simulink model "BLAC_MotorCtrl_Math"  (R2025b)
settings: Solver=FixedStepDiscrete  StartTime=0.0  StopTime=5  FixedStep=MC_Sim_BaseStep  RelTol=1e-3  EnableMultiTasking=on
values from neighbouring files (symbols this model uses):
  MC_Hardware_Chip_ADCResultBit = 0.0    [MotorControlDataDictionary_Math.sldd]
  MC_Hardware_Chip_ADCVoltageMax = 1.0    [MotorControlDataDictionary_Math.sldd]
  MC_Hardware_Chip_ADCVoltageRefence = 0.0    [MotorControlDataDictionary_Math.sldd]
  MC_Hardware_Chip_CSAGain = 1.0    [MotorControlDataDictionary_Math.sldd]
  MC_Sim_BaseStep = 2.5E-8    [MotorControlDataDictionary_Math.sldd]
  MC_Sim_HFTStep = 6.6675E-5    [MotorControlDataDictionary_Math.sldd]
undefined symbols (not defined in the file or in its folder): MC_MOS_DeadTime, MC_Motor_Phi, MC_Motor_Rotor_Pn, MC_Motor_Stator_Ld, MC_Motor_Stator_Lq, MC_Motor_Stator_Rs, MC_Param_CurrentPI_Ki, MC_Param_CurrentPI_Kp, MC_Param_CurrentPI_UdInteMax, MC_Param_CurrentPI_UdInteMin, MC_Param_CurrentPI_UdMax, MC_Param_CurrentPI_UdMin, MC_Param_CurrentPI_UqInteMax, MC_Param_CurrentPI_UqInteMin, MC_Param_CurrentPI_UqMax, MC_Param_CurrentPI_UqMin, MC_Param_Flux_Gamma, MC_Param_Flux_Lalpha, MC_Param_Flux_Lbeta, MC_Param_Flux_Ralpha, MC_Param_Flux_Rbeta, MC_Param_Luen_BEMFalpha, MC_Param_Luen_BEMFbeta, MC_Param_Luen_BEMFErr, MC_Param_Luen_Currentalpha, MC_Param_Luen_Currentbeta, MC_Param_Luen_CurrentErr, MC_Param_Luen_PLL_Ki, MC_Param_Luen_PLL_Kp, MC_Param_Luen_Voltagealpha, MC_Param_Luen_Voltagebeta, MC_Param_PhasetoReal, MC_Param_SMO_CoffA, MC_Param_SMO_CoffB, MC_Param_SpeedtoTheta, MC_Param_SVPWM_DutyMax, MC_Param_SVPWM_DutyMin, MC_Param_SVPWM_SampleOffset1, MC_Param_SVPWM_SampleOffset2, MC_Param_SVPWM_SampleValid
libraries: simulink x31, nesl_utility x22, ee_lib x21, fl_lib x16, spsSeriesRLCBranchLib x2, spsVoltageMeasurementLib x2
(part 4 of 5)

== system BLAC_MotorCtrl_Math/HFTask/fluxobservor/getFlux ==
  note: 日志：
      | 2025.02.28：滑膜观测器建模无问题，但是反电势观测存在问题，暂时分析为参数问题
  Valpha : Inport
  Vbeta : Inport  Port=2
  Ialpha : Inport  Port=3
  Ibeta : Inport  Port=4
  Add{,1..4} (5 alike) : Sum
  Constant : Constant  Value=MC_Motor_Phi  OutDataTypeStr=single
  Delay One Step{,1..3} (4 alike) : Delay  DelayLength=1
  Gain : Gain  Gain=MC_Param_Flux_Ralpha
  Gain1 : Gain  Gain=MC_Param_Flux_Gamma  OutDataTypeStr=single  RndMeth=Simplest
  Gain2 : Gain  Gain=single(MC_Sim_HFTStep)  OutDataTypeStr=single  RndMeth=Simplest
  Gain3 : Gain  Gain=MC_Param_Flux_Lalpha  OutDataTypeStr=single  RndMeth=Simplest
  Gain4 : Gain  Gain=MC_Param_Flux_Rbeta
  Gain5 : Gain  Gain=MC_Param_Flux_Gamma  OutDataTypeStr=single  RndMeth=Simplest
  Gain6 : Gain  Gain=single(MC_Sim_HFTStep)
  Gain7 : Gain  Gain=MC_Param_Flux_Lbeta  OutDataTypeStr=single  RndMeth=Simplest
  Product : Product
  Product1 : Product
  Square : Math  Operator=square
  Square1 : Math  Operator=square
  Square2 : Math  Operator=square
  Subtract{,1..4} (5 alike) : Sum  Inputs=+-
  Phialpha : Outport
  Phibeta : Outport  Port=2
  wires:
  Valpha/1 -> Subtract/1
  Ialpha/1 -> Gain3/1, Gain/1
  Gain/1 -> Subtract/2
  Subtract/1 -> Add/1  "Y_Alpha"
  Gain1/1 -> Add/2  "NLFcn_Alpha"
  Add/1 -> Gain2/1  "Xdot_Alpha"
  Add1/1 -> Subtract1/1, Delay One Step/1  "X_Alpha"
  Delay One Step/1 -> Add1/2
  Gain2/1 -> Add1/1
  Gain3/1 -> Subtract1/2
  Subtract1/1 -> Phialpha/1, Delay One Step1/1  "Phialpha"
  Product/1 -> Gain1/1
  Delay One Step1/1 -> [Nx_alpha], Product/2
  Delay One Step3/1 -> [Nx_beta], Product1/2
  Product1/1 -> Gain5/1
  Subtract3/1 -> Phibeta/1, Delay One Step3/1  "Phibeta"
  Gain7/1 -> Subtract3/2
  Gain6/1 -> Add3/1
  Delay One Step2/1 -> Add3/2
  Add3/1 -> Delay One Step2/1, Subtract3/1  "X_Beta"
  Add2/1 -> Gain6/1  "Xdot_Beta"
  Gain5/1 -> Add2/2  "NLFcn_Beta"
  Subtract2/1 -> Add2/1  "Y_Beta"
  Gain4/1 -> Subtract2/2
  Ibeta/1 -> Gain4/1, Gain7/1
  Vbeta/1 -> Subtract2/1
  Constant/1 -> Square/1
  [Nx_alpha] -> Square1/1
  [Nx_beta] -> Square2/1
  Square1/1 -> Add4/1
  Square2/1 -> Add4/2
  Square/1 -> Subtract4/1
  Add4/1 -> Subtract4/2  "Psim2"
  Subtract4/1 -> [Nx2]  "Nx2"
  [Nx2] -> Product/1
  [Nx2] -> Product1/1

== system BLAC_MotorCtrl_Math/HFTask/fluxobservor/getSpeedandTheta ==
  Phialpha : Inport
  Phibeta : Inport  Port=2
  Add : Sum
  Add1 : Sum
  Add2 : Sum
  Constant : Constant  Value=2*pi  OutDataTypeStr=single
  Delay One Step : Delay  DelayLength=1
  Delay One Step2 : Delay  DelayLength=1
  Gain : Gain  Gain=1/MC_Motor_Phi
  Gain1 : Gain  Gain=2*sqrt(2)/2*100
  Gain2 : Gain  Gain=100^2*MC_Sim_HFTStep
  Gain3 : Gain  Gain=MC_Param_SpeedtoTheta  OutDataTypeStr=single  RndMeth=Simplest
  Gain4 : Gain  Gain=1/MC_Motor_Phi
  Gain5 : Gain  Gain=30/(pi*MC_Motor_Rotor_Pn)  OutDataTypeStr=single  RndMeth=Simplest
  Mod : Math  Operator=mod
  Product : Product
  Product1 : Product
  Sin : Trigonometry  OutputSignalType=real
  Sin1 : Trigonometry  Operator=cos  OutputSignalType=real
  Subtract : Sum  Inputs=+-
  Speed : Outport
  Theta : Outport  Port=2
  wires:
  [Theta_Last] -> Sin/1, Sin1/1
  Add1/1 -> Gain5/1, Gain3/1  "WeFlux"
  Mod/1 -> Delay One Step2/1, Theta/1  "ThetaFlux"
  Delay One Step2/1 -> [Theta_Last], Add2/2
  Constant/1 -> Mod/2
  Add2/1 -> Mod/1
  Gain3/1 -> Add2/1
  Subtract/1 -> Gain1/1, Gain2/1  "FluxErr"
  Gain1/1 -> Add1/1
  Delay One Step/1 -> Add/2
  Add/1 -> Add1/2, Delay One Step/1
  Gain2/1 -> Add/1
  Product1/1 -> Subtract/2  "FluxSin"
  Product/1 -> Subtract/1  "FluxCos"
  Sin/1 -> Product1/2
  Sin1/1 -> Product/2
  Phibeta/1 -> Gain/1
  Phialpha/1 -> Gain4/1
  Gain/1 -> Product/1
  Gain4/1 -> Product1/1
  Gain5/1 -> Speed/1  "SpeedFlux_RPM"

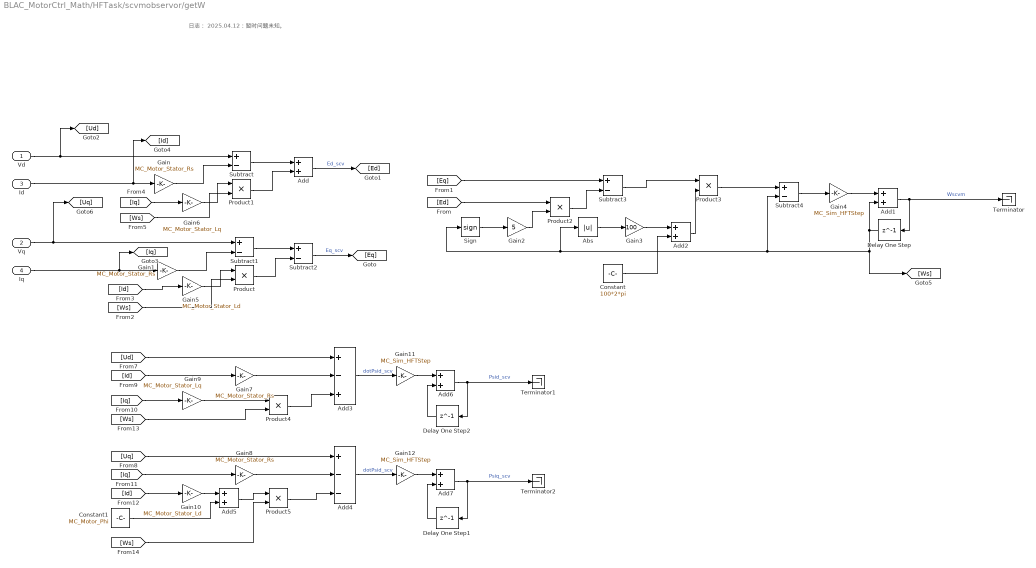
== system BLAC_MotorCtrl_Math/HFTask/scvmobservor/getW ==
  note: 日志：
      | 2025.04.12：暂时问题未知。
  Vd : Inport
  Vq : Inport  Port=2
  Id : Inport  Port=3
  Iq : Inport  Port=4
  Abs : Abs  SaturateOnIntegerOverflow=off
  Add{,1..2,5..7} (6 alike) : Sum
  Add3 : Sum  Inputs=+-+
  Add4 : Sum  Inputs=+--
  Constant : Constant  Value=100*2*pi  OutDataTypeStr=single
  Constant1 : Constant  Value=MC_Motor_Phi  OutDataTypeStr=single
  Delay One Step : Delay  DelayLength=1
  Delay One Step1 : Delay  DelayLength=1
  Delay One Step2 : Delay  DelayLength=1
  Gain{,1,7..8} (4 alike) : Gain  Gain=MC_Motor_Stator_Rs
  Gain10 : Gain  Gain=MC_Motor_Stator_Ld
  Gain11 : Gain  Gain=MC_Sim_HFTStep
  Gain12 : Gain  Gain=MC_Sim_HFTStep
  Gain2 : Gain  Gain=5
  Gain3 : Gain  Gain=100
  Gain4 : Gain  Gain=MC_Sim_HFTStep
  Gain5 : Gain  Gain=MC_Motor_Stator_Ld
  Gain6 : Gain  Gain=MC_Motor_Stator_Lq
  Gain9 : Gain  Gain=MC_Motor_Stator_Lq
  Product{,1..5} (6 alike) : Product
  Sign : Signum
  Subtract{,1..4} (5 alike) : Sum  Inputs=+-
  Terminator : Terminator
  Terminator1 : Terminator
  Terminator2 : Terminator
  wires:
  Id/1 -> [Id], Gain/1
  Gain/1 -> Subtract/2
  Subtract/1 -> Add/1
  Add/1 -> [Ed]  "Ed_scv"
  Gain1/1 -> Subtract1/2
  Iq/1 -> [Iq], Gain1/1
  Vq/1 -> Subtract1/1, [Uq]
  Subtract1/1 -> Subtract2/1
  Product/1 -> Subtract2/2
  Product1/1 -> Add/2
  Subtract2/1 -> [Eq]  "Eq_scv"
  [Ed] -> Product2/1
  Gain2/1 -> Product2/2
  Sign/1 -> Gain2/1
  [Eq] -> Subtract3/1
  Product2/1 -> Subtract3/2
  Subtract3/1 -> Product3/1
  Product3/1 -> Subtract4/1
  Gain4/1 -> Add1/1
  Add1/1 -> Delay One Step/1, Terminator/1  "Wscvm"
  Delay One Step/1 -> [Ws], Subtract4/2, Abs/1, Sign/1, Add1/2
  Subtract4/1 -> Gain4/1
  [Id] -> Gain5/1
  Gain5/1 -> Product/1
  [Ws] -> Product/2
  Gain6/1 -> Product1/1
  [Iq] -> Gain6/1
  [Ws] -> Product1/2
  Abs/1 -> Gain3/1
  Add2/1 -> Product3/2
  Gain3/1 -> Add2/1
  Constant/1 -> Add2/2
  Vd/1 -> Subtract/1, [Ud]
  [Id] -> Gain7/1
  [Iq] -> Gain8/1
  [Ud] -> Add3/1
  Gain7/1 -> Add3/2
  Gain8/1 -> Add4/2
  [Uq] -> Add4/1
  [Ws] -> Product4/2
  Product4/1 -> Add3/3
  Product5/1 -> Add4/3
  [Iq] -> Gain9/1
  Gain9/1 -> Product4/1
  [Id] -> Gain10/1
  Gain10/1 -> Add5/1
  Constant1/1 -> Add5/2
  Add5/1 -> Product5/1
  [Ws] -> Product5/2
  Add3/1 -> Gain11/1  "dotPsid_scv"
  Add4/1 -> Gain12/1  "dotPsid_scv"
  Add7/1 -> Terminator2/1, Delay One Step1/1  "Psiq_scv"
  Delay One Step1/1 -> Add7/2
  Add6/1 -> Terminator1/1, Delay One Step2/1  "Psid_scv"
  Delay One Step2/1 -> Add6/2
  Gain11/1 -> Add6/1
  Gain12/1 -> Add7/1

== system BLAC_MotorCtrl_Math/HFTask/smo/getE ==
  note: 日志：
      | 2025.02.28：滑膜观测器建模无问题，但是反电势观测存在问题，暂时分析为参数问题
  Valpha : Inport
  Vbeta : Inport  Port=2
  Ialpha : Inport  Port=3
  Ibeta : Inport  Port=4
  Add : Sum  Inputs=--+
  Add1 : Sum
  Add2 : Sum  Inputs=+--
  Add3 : Sum
  Delay One Step{,1..3} (4 alike) : Delay  DelayLength=1
  Gain{,4,6,8} (4 alike) : Gain  Gain=MC_Param_SMO_CoffB
  Gain3 : Gain  Gain=MC_Param_SMO_CoffA
  Gain7 : Gain  Gain=MC_Param_SMO_CoffA
  Saturation : Saturate  UpperLimit=100  LowerLimit=-100
  Saturation1 : Saturate  UpperLimit=100  LowerLimit=-100
  Subtract : Sum  Inputs=+-
  Subtract1 : Sum  Inputs=-+
  Ealpha : Outport
  Ebeta : Outport  Port=2
  wires:
  Valpha/1 -> Gain/1
  Add1/1 -> Subtract/1, Delay One Step/1  "Ialpha_SMO"
  Ialpha/1 -> Subtract/2
  Gain/1 -> Add/3
  Gain3/1 -> Add/2
  Gain4/1 -> Add/1
  Delay One Step1/1 -> [Ealpha_SMO]
  [Ialpha_SMO] -> Gain3/1
  [Ealpha_SMO] -> Gain4/1
  Subtract/1 -> Saturation/1
  Saturation/1 -> Ealpha/1, Delay One Step1/1  "Ealpha_SMO"
  Gain6/1 -> Add2/1
  Gain7/1 -> Add2/2
  Gain8/1 -> Add2/3
  Vbeta/1 -> Gain6/1
  Add/1 -> Add1/1  "dotIalpha_SMO"
  Delay One Step/1 -> Add1/2, [Ialpha_SMO]
  Add2/1 -> Add3/2  "dotIbeta_SMO"
  Add3/1 -> Subtract1/2, Delay One Step2/1  "Ibeta_SMO"
  Delay One Step2/1 -> [Ibeta_SMO], Add3/1
  Ibeta/1 -> Subtract1/1
  Subtract1/1 -> Saturation1/1
  Saturation1/1 -> Ebeta/1, Delay One Step3/1  "Ebeta_SMO"
  Delay One Step3/1 -> [Ebeta_SMO]
  [Ibeta_SMO] -> Gain7/1
  [Ebeta_SMO] -> Gain8/1

== system BLAC_MotorCtrl_Math/HFTask/smo/getSpeedandTheta ==
  note: 日志：
      | 2025.03.19：反电势正负号识别错误，改正后可以使用
  Ealpha : Inport
  Ebeta : Inport  Port=2
  Add : Sum
  Add1 : Sum
  Add2 : Sum
  Constant : Constant  Value=2*pi  OutDataTypeStr=single
  Delay One Step : Delay  DelayLength=1
  Delay One Step2 : Delay  DelayLength=1
  Gain : Gain  Gain=-1
  Gain1 : Gain  Gain=2*sqrt(2)/2*100
  Gain2 : Gain  Gain=100^2*MC_Sim_HFTStep
  Gain3 : Gain  Gain=MC_Param_SpeedtoTheta
  Gain5 : Gain  Gain=30/(pi*MC_Motor_Rotor_Pn)  OutDataTypeStr=single  RndMeth=Simplest
  Mod : Math  Operator=mod
  Product : Product
  Product1 : Product
  Sin : Trigonometry  OutputSignalType=real
  Sin1 : Trigonometry  Operator=cos  OutputSignalType=real
  Subtract : Sum  Inputs=+-
  Speed : Outport
  Theta : Outport  Port=2
  wires:
  Sin1/1 -> Product/2
  Sin/1 -> Product1/2
  Gain2/1 -> Add/1
  Add/1 -> Delay One Step/1, Add1/2
  Delay One Step/1 -> Add/2
  Gain1/1 -> Add1/1
  Subtract/1 -> Gain2/1, Gain1/1  "SMOErr"
  Gain3/1 -> Add2/1
  Add2/1 -> Mod/1
  Constant/1 -> Mod/2
  Delay One Step2/1 -> Add2/2, [Theta_Last]
  Mod/1 -> Theta/1, Delay One Step2/1  "ThetaSMO"
  Add1/1 -> Gain5/1, Gain3/1  "SpeedSmo"
  [Theta_Last] -> Sin1/1, Sin/1
  Gain/1 -> Product1/1
  Ebeta/1 -> Gain/1
  Ealpha/1 -> Product/1
  Product/1 -> Subtract/1  "SMOSin"
  Product1/1 -> Subtract/2  "SMOCos"
  Gain5/1 -> Speed/1  "SpeedSMO_RPM"

== system BLAC_MotorCtrl_Math/HFTask/svpwm/getVoltageExchange ==
  Valpha : Inport
  Vbeta : Inport  Port=2
  Vdc : Inport  Port=3
  Add : Sum
  Add1 : Sum
  Divide : Product  Inputs=*/
  Divide1 : Product  Inputs=*/
  Gain : Gain  Gain=-1/2
  Gain1 : Gain  Gain=sqrt(3)/2
  Gain2 : Gain  Gain=-1
  Relational Operator : RelationalOperator  OutDataTypeStr=boolean  RndMeth=Simplest  InputSameDT=off
  Relational Operator1 : RelationalOperator  OutDataTypeStr=boolean  RndMeth=Simplest  InputSameDT=off
  Relational Operator2 : RelationalOperator  Operator=<=  OutDataTypeStr=boolean  RndMeth=Simplest  InputSameDT=off
  Relational Operator3 : RelationalOperator  Operator=<=  OutDataTypeStr=boolean  RndMeth=Simplest  InputSameDT=off
  Signal Copy : SignalConversion  OverrideOpt=off
  Subtract : Sum  Inputs=+-
  Switch{,1..3} (4 alike) : Switch  Criteria=u2 > Threshold  SaturateOnIntegerOverflow=off  InputSameDT=off
  getSectorN : Subsystem  Commented=on
  Va : Outport
  Vb : Outport  Port=2
  Vc : Outport  Port=3
  Vmed : Outport  Port=4
  wires:
  Valpha/1 -> Divide/1
  Vbeta/1 -> Divide1/1
  Vdc/1 -> Divide/2, Divide1/2
  Subtract/1 -> Relational Operator3/2, Switch3/3, Relational Operator1/2, Switch1/3, Vc/1  "Vc"
  Add/1 -> Switch2/3, Relational Operator2/2, Switch/3, Relational Operator/2, Vb/1  "Vb"
  Gain1/1 -> Subtract/2, Add/2
  Gain/1 -> Add/1, Subtract/1
  Divide1/1 -> Gain1/1
  Divide/1 -> Gain/1, Signal Copy/1
  Signal Copy/1 -> Switch2/1, Relational Operator2/1, Switch/1, Relational Operator/1, Va/1  "Va"
  Switch1/1 -> Add1/1  "Vmax"
  Relational Operator1/1 -> Switch1/2
  Switch/1 -> Relational Operator1/1, Switch1/1
  Relational Operator/1 -> Switch/2
  Switch3/1 -> Add1/2  "Vmin"
  Relational Operator3/1 -> Switch3/2
  Switch2/1 -> Switch3/1, Relational Operator3/1
  Relational Operator2/1 -> Switch2/2
  Add1/1 -> Gain2/1
  Gain2/1 -> Vmed/1  "Vmed"

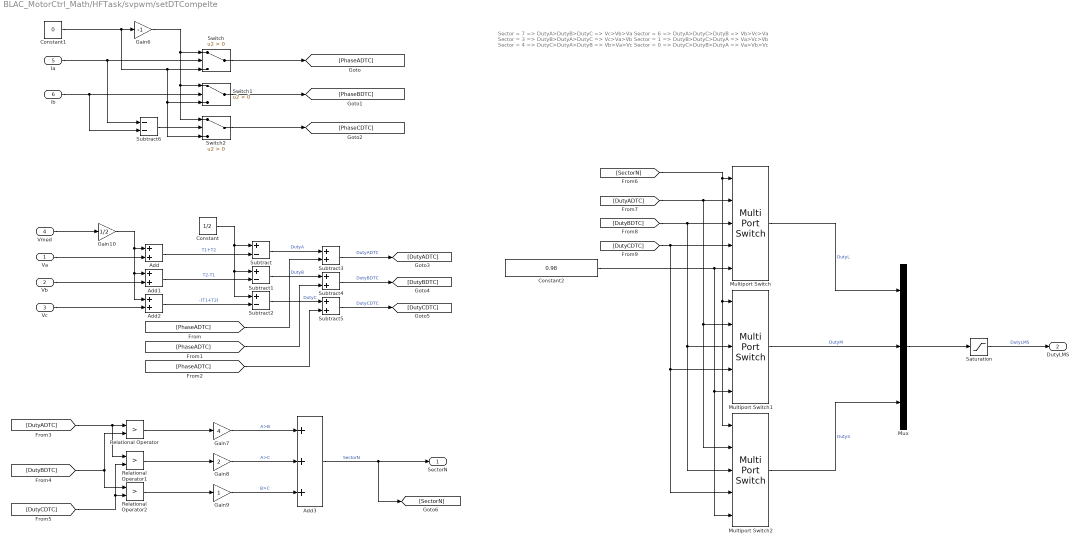
== system BLAC_MotorCtrl_Math/HFTask/svpwm/setDTCompelte ==
  note: Sector = 7 => DutyA>DutyB>DutyC => Vc>Vb>Va
      | Sector = 6 => DutyA>DutyC>DutyB => Vb>Vc>Va
      | Sector = 3 => DutyB>DutyA>DutyC => Vc>Va>Vb
      | Sector = 1 => DutyB>DutyC>DutyA => Va>Vc>Vb
      | Sector = 4 => DutyC>DutyA>DutyB => Vb>Va>Vc
      | Sector = 0 => DutyC>DutyB>DutyA => Va>Vb>Vc
  Va : Inport
  Vb : Inport  Port=2
  Vc : Inport  Port=3
  Vmed : Inport  Port=4
  Ia : Inport  Port=5
  ib : Inport  Port=6
  Add : Sum
  Add1 : Sum
  Add2 : Sum
  Add3 : Sum  Inputs=+++
  Constant : Constant  Value=1/2  OutDataTypeStr=single  SampleTime=MC_Sim_HFTStep
  Constant1 : Constant  Value=0  OutDataTypeStr=single
  Constant2 : Constant  Value=0.98  OutDataTypeStr=single
  Gain10 : Gain  Gain=1/2
  Gain6 : Gain  Gain=-1
  Gain7 : Gain  Gain=4  OutDataTypeStr=single  RndMeth=Simplest
  Gain8 : Gain  Gain=2  OutDataTypeStr=single  RndMeth=Simplest
  Gain9 : Gain  OutDataTypeStr=single  RndMeth=Simplest
  Multiport Switch : MultiPortSwitch  DataPortOrder=Specify indices  DataPortIndices={[6,7],[1,3],[0,4]}  DataPortForDefault=Additional data port  SaturateOnIntegerOverflow=off  InputSameDT=off
  Multiport Switch1 : MultiPortSwitch  DataPortOrder=Specify indices  DataPortIndices={[4,3],[7,0],[6,1]}  DataPortForDefault=Additional data port  SaturateOnIntegerOverflow=off  InputSameDT=off
  Multiport Switch2 : MultiPortSwitch  DataPortOrder=Specify indices  DataPortIndices={[0,1],[4,6],[3,7]}  DataPortForDefault=Additional data port  SaturateOnIntegerOverflow=off  InputSameDT=off
  Mux : Mux  Inputs=3
  Relational Operator : RelationalOperator  Operator=>  OutDataTypeStr=boolean  RndMeth=Simplest  InputSameDT=off
  Relational Operator1 : RelationalOperator  Operator=>  OutDataTypeStr=boolean  RndMeth=Simplest  InputSameDT=off
  Relational Operator2 : RelationalOperator  Operator=>  OutDataTypeStr=boolean  RndMeth=Simplest  InputSameDT=off
  Saturation : Saturate  UpperLimit=0.98  LowerLimit=0.02
      settings: AttributesFormatString=|
      | OutputMax = %<UpperLimit>
      | OutputMin = %<LowerLimit>
  Subtract : Sum  Inputs=+-
  Subtract1 : Sum  Inputs=+-
  Subtract2 : Sum  Inputs=+-
  Subtract3 : Sum
  Subtract4 : Sum
  Subtract5 : Sum
  Subtract6 : Sum  Inputs=--
  Switch : Switch  Criteria=u2 > Threshold  SaturateOnIntegerOverflow=off  InputSameDT=off
  Switch1 : Switch  Criteria=u2 > Threshold  SaturateOnIntegerOverflow=off  InputSameDT=off
  Switch2 : Switch  Criteria=u2 > Threshold  SaturateOnIntegerOverflow=off  InputSameDT=off
  SectorN : Outport
  DutyLMS : Outport  Port=2
  wires:
  Va/1 -> Add/2
  Vmed/1 -> Gain10/1
  Vb/1 -> Add1/2
  Vc/1 -> Add2/2
  Add/1 -> Subtract/2  "T1+T2"
  Add2/1 -> Subtract2/2  "-(T1+T2)"
  Add1/1 -> Subtract1/2  "T2-T1"
  Constant/1 -> Subtract2/1, Subtract1/1, Subtract/1
  Subtract/1 -> Subtract3/1  "DutyA"
  Subtract1/1 -> Subtract4/1  "DutyB"
  Subtract2/1 -> Subtract5/1  "DutyC"
  Ia/1 -> Subtract6/1, Switch/2
  Gain6/1 -> Switch2/1, Switch1/1, Switch/1
  ib/1 -> Subtract6/2, Switch1/2
  Subtract6/1 -> Switch2/2
  Constant1/1 -> Switch2/3, Switch1/3, Switch/3, Gain6/1
  Switch/1 -> [PhaseADTC]
  Switch1/1 -> [PhaseBDTC]
  Switch2/1 -> [PhaseCDTC]
  [PhaseADTC] -> Subtract3/2
  [PhaseADTC] -> Subtract4/2
  [PhaseADTC] -> Subtract5/2
  [DutyBDTC] -> Relational Operator/2, Relational Operator2/1
  [DutyADTC] -> Relational Operator1/1, Relational Operator/1
  [DutyCDTC] -> Relational Operator2/2, Relational Operator1/2
  Relational Operator/1 -> Gain7/1
  Relational Operator1/1 -> Gain8/1
  Relational Operator2/1 -> Gain9/1
  Gain8/1 -> Add3/2  "A>C"
  Gain9/1 -> Add3/3  "B>C"
  Gain7/1 -> Add3/1  "A>B"
  Add3/1 -> [SectorN], SectorN/1  "SectorN"
  Gain10/1 -> Add2/1, Add1/1, Add/1
  Subtract3/1 -> [DutyADTC]  "DutyADTC"
  Subtract4/1 -> [DutyBDTC]  "DutyBDTC"
  Subtract5/1 -> [DutyCDTC]  "DutyCDTC"
  [SectorN] -> Multiport Switch2/1, Multiport Switch1/1, Multiport Switch/1
  Multiport Switch/1 -> Mux/1  "DutyL"
  Constant2/1 -> Multiport Switch2/5, Multiport Switch1/5, Multiport Switch/5
  Multiport Switch1/1 -> Mux/2  "DutyM"
  Multiport Switch2/1 -> Mux/3  "DutyS"
  Mux/1 -> Saturation/1
  Saturation/1 -> DutyLMS/1  "DutyLMS"
  [DutyADTC] -> Multiport Switch2/2, Multiport Switch1/2, Multiport Switch/2
  [DutyCDTC] -> Multiport Switch2/4, Multiport Switch1/4, Multiport Switch/4
  [DutyBDTC] -> Multiport Switch2/3, Multiport Switch1/3, Multiport Switch/3

== system BLAC_MotorCtrl_Math/HFTask/svpwm/setPhaseandSample_ORS_Double ==
  note: 电流采样方案：
      | 1、电压满足采样时间，直接计算电流采样点，采样点有效
      | 2、周期内总电压满足采样时间，
  note: Sector = 7 => DutyA>DutyB>DutyC => Vc>Vb>Va
      | Sector = 6 => DutyA>DutyC>DutyB => Vb>Vc>Va
      | Sector = 3 => DutyB>DutyA>DutyC => Vc>Va>Vb
      | Sector = 1 => DutyB>DutyC>DutyA => Va>Vc>Vb
      | Sector = 4 => DutyC>DutyA>DutyB => Vb>Va>Vc
      | Sector = 0 => DutyC>DutyB>DutyA => Va>Vb>Vc
  SectorN : Inport
  DutyLMS : Inport  Port=2
  Constant{1,4,6..8} (5 alike) : Constant  OutDataTypeStr=single
  Constant2 : Constant  Value=boolean(1)  OutDataTypeStr=single
  Constant3 : Constant  Value=boolean(1)  OutDataTypeStr=single
  Constant5 : Constant  Value=0.98  OutDataTypeStr=single
  Demux : Demux  Outputs=3
  Multiport Switch : MultiPortSwitch  DataPortOrder=Specify indices  DataPortIndices={[7,6],[3,4],[0,1]}  DataPortForDefault=Additional data port  SaturateOnIntegerOverflow=off  InputSameDT=off
  Multiport Switch1 : MultiPortSwitch  DataPortOrder=Specify indices  DataPortIndices={[3,1],[7,0],[6,4]}  DataPortForDefault=Additional data port  SaturateOnIntegerOverflow=off  InputSameDT=off
  Multiport Switch2 : MultiPortSwitch  DataPortOrder=Specify indices  DataPortIndices={[4,0],[6,1],[7,3]}  DataPortForDefault=Additional data port  SaturateOnIntegerOverflow=off  InputSameDT=off
  Mux : Mux  Inputs=2
  Mux1 : Mux  Inputs=5
  Mux2 : Mux  Inputs=2
  Mux5 : Mux  Inputs=3
  Saturation : Saturate  UpperLimit=0.98  LowerLimit=0.02
      settings: AttributesFormatString=|
      | OutputMax = %<UpperLimit>
      | OutputMin = %<LowerLimit>
  Subtract : Sum  Inputs=+-
  Subtract1 : Sum  Inputs=+-
  DutySVPWM : Outport
  SamplePoint : Outport  Port=2
  SampleValid : Outport  Port=3
  wires:
  DutyLMS/1 -> Demux/1
  Subtract/1 -> [T1divid2]  "T1/2"
  Subtract1/1 -> [T2divid2]  "T2/2"
  SectorN/1 -> [SectorN]
  [SectorN] -> Multiport Switch2/1, Multiport Switch1/1, Multiport Switch/1
  [DutyLPM] -> Multiport Switch2/2, Multiport Switch1/2, Multiport Switch/2
  [DutyMPM] -> Multiport Switch2/3, Multiport Switch1/3, Multiport Switch/3
  [DutySPM] -> Multiport Switch1/4, Multiport Switch2/4, Multiport Switch/4
  Constant5/1 -> Multiport Switch1/5, Multiport Switch/5, Multiport Switch2/5
  Multiport Switch1/1 -> Mux5/2  "DutyBPM[2]"
  Multiport Switch2/1 -> Mux5/3  "DutyCPM[2]"
  Multiport Switch/1 -> Mux5/1  "DutyAPM[2]"
  Saturation/1 -> DutySVPWM/1  "DutySVPWM[6]"
  Demux/1 -> [DutyL], Subtract1/1
  Demux/2 -> [DutyM], Subtract1/2, Subtract/1
  Demux/3 -> Subtract/2, [DutyS]
  Constant2/1 -> Mux/1
  Constant3/1 -> Mux/2
  Mux/1 -> SampleValid/1
  Constant4/1 -> Mux1/2
  Constant1/1 -> Mux1/1
  Mux1/1 -> SamplePoint/1
  Constant6/1 -> Mux1/3
  Constant8/1 -> Mux1/4
  Constant7/1 -> Mux1/5
  Mux5/1 -> Mux2/2, Mux2/1
  Mux2/1 -> Saturation/1

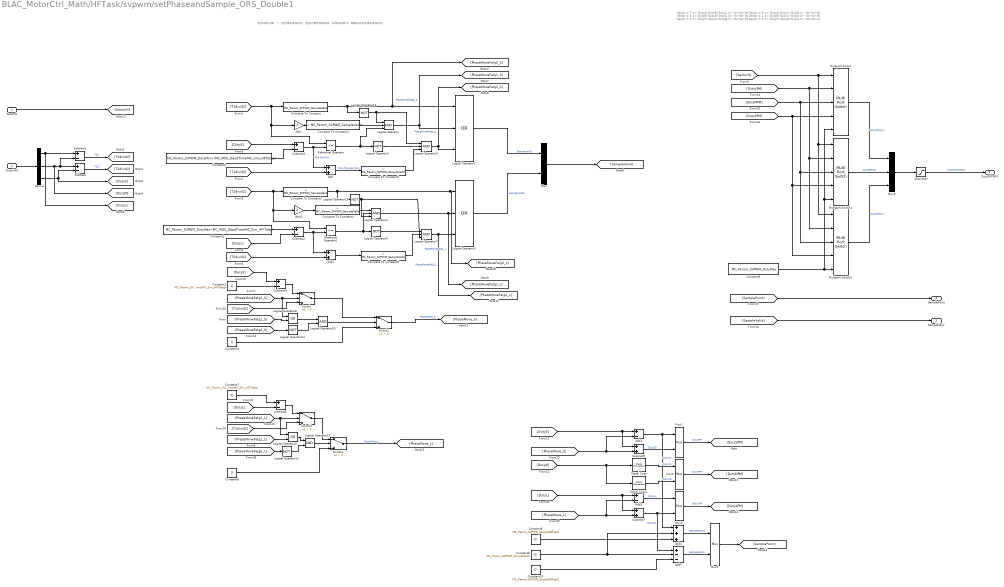
== system BLAC_MotorCtrl_Math/HFTask/svpwm/setPhaseandSample_ORS_Double1 ==
  note: Sector = 7 => DutyA>DutyB>DutyC => Vc>Vb>Va
      | Sector = 6 => DutyA>DutyC>DutyB => Vb>Vc>Va
      | Sector = 3 => DutyB>DutyA>DutyC => Vc>Va>Vb
      | Sector = 1 => DutyB>DutyC>DutyA => Va>Vc>Vb
      | Sector = 4 => DutyC>DutyA>DutyB => Vb>Va>Vc
      | Sector = 0 => DutyC>DutyB>DutyA => Va>Vb>Vc
  note: 电流采样方案：
      | 1、电压满足采样时间，直接计算电流采样点，采样点有效
      | 2、周期内总电压满足采样时间，
  SectorN : Inport
  DutyLMS : Inport  Port=2
  Add : Sum
  Add1 : Sum
  Add2 : Sum  Inputs=+-
  Add3 : Sum  Inputs=+-
  Add4 : Sum  Inputs=+++
  Add5 : Sum  Inputs=+--
  Compare To Constant{,1..5} (6 alike) : simulink/Logic and Bit Operations/Compare To Constant  relop=>  const=MC_Param_SVPWM_SampleValid  OutDataTypeStr=boolean
  Constant1 : Constant  Value=MC_Param_SVPWM_DutyMax-(MC_MOS_DeadTime/MC_Sim_HFTStep)  OutDataTypeStr=single
  Constant10 : Constant  Value=MC_Param_SVPWM_SampleOffset2  OutDataTypeStr=single
  Constant2 : Constant  Value=MC_Param_SVPWM_DutyMin+(MC_MOS_DeadTime/MC_Sim_HFTStep)  OutDataTypeStr=single
  Constant3 : Constant  Value=MC_Param_SVPWM_DutyMin+(MC_MOS_DeadTime/MC_Sim_HFTStep)  OutDataTypeStr=single
  Constant4 : Constant  Value=0  OutDataTypeStr=single
  Constant5 : Constant  Value=MC_Param_SVPWM_DutyMax  OutDataTypeStr=single
  Constant6 : Constant  Value=0  OutDataTypeStr=single
  Constant7 : Constant  Value=MC_Param_SVPWM_DutyMax-(MC_MOS_DeadTime/MC_Sim_HFTStep)  OutDataTypeStr=single
  Constant8 : Constant  Value=MC_Param_SVPWM_SampleValid  OutDataTypeStr=single
  Constant9 : Constant  Value=MC_Param_SVPWM_SampleOffset1  OutDataTypeStr=single
  Demux : Demux  Outputs=3
  Gain : Gain  Gain=2
  Gain1 : Gain  Gain=2
  Logical Operator{,3..4,7} (4 alike) : Logic  Inputs=3  AllPortsSameDT=off  OutDataTypeStr=boolean
  Logical Operator1 : Logic  Operator=OR  Inputs=3  AllPortsSameDT=off  OutDataTypeStr=boolean
  Logical Operator10 : Logic  AllPortsSameDT=off  OutDataTypeStr=boolean
  Logical Operator{2,6,11..12,14..15} (6 alike) : Logic  Operator=NOT  AllPortsSameDT=off  OutDataTypeStr=boolean
  Logical Operator13 : Logic  AllPortsSameDT=off  OutDataTypeStr=boolean
  Logical Operator5 : Logic  Operator=OR  Inputs=3  AllPortsSameDT=off  OutDataTypeStr=boolean
  Logical Operator8 : Logic  Operator=OR  AllPortsSameDT=off  OutDataTypeStr=boolean
  Logical Operator9 : Logic  Operator=OR  AllPortsSameDT=off  OutDataTypeStr=boolean
  Multiport Switch : MultiPortSwitch  DataPortOrder=Specify indices  DataPortIndices={[7,6],[3,4],[0,1]}  DataPortForDefault=Additional data port  SaturateOnIntegerOverflow=off  InputSameDT=off
  Multiport Switch1 : MultiPortSwitch  DataPortOrder=Specify indices  DataPortIndices={[3,1],[7,0],[6,4]}  DataPortForDefault=Additional data port  SaturateOnIntegerOverflow=off  InputSameDT=off
  Multiport Switch2 : MultiPortSwitch  DataPortOrder=Specify indices  DataPortIndices={[4,0],[6,1],[7,3]}  DataPortForDefault=Additional data port  SaturateOnIntegerOverflow=off  InputSameDT=off
  Mux{,1..4} (5 alike) : Mux  Inputs=2
  Mux5 : Mux  Inputs=3
  Relational Operator : RelationalOperator  Operator=<=  OutDataTypeStr=boolean  RndMeth=Simplest  InputSameDT=off
  Relational Operator1 : RelationalOperator  Operator=<=  OutDataTypeStr=boolean  RndMeth=Simplest  InputSameDT=off
  Saturation : Saturate  UpperLimit=MC_Param_SVPWM_DutyMax  LowerLimit=MC_Param_SVPWM_DutyMin
      settings: AttributesFormatString=|
      | OutputMax = %<UpperLimit>
      | OutputMin = %<LowerLimit>
  Signal Copy : SignalConversion  OverrideOpt=off
  Signal Copy1 : SignalConversion  OverrideOpt=off
  Subtract{,1..4,6} (6 alike) : Sum  Inputs=+-
  Subtract5 : Sum
  Subtract7 : Sum
  Switch{,1..3} (4 alike) : Switch  Criteria=u2 > Threshold  SaturateOnIntegerOverflow=off  InputSameDT=off
  DutySVPWM : Outport
  SamplePoint : Outport  Port=2
  SampleValid : Outport  Port=3
  wires:
  Logical Operator15/1 -> Logical Operator7/3, Logical Operator4/3
  Compare To Constant2/1 -> Logical Operator3/3
  Logical Operator2/1 -> Logical Operator3/2
  Logical Operator14/1 -> Logical Operator/1, Logical Operator3/1
  Compare To Constant1/1 -> Logical Operator/2
  Logical Operator12/1 -> Logical Operator13/2
  Logical Operator9/1 -> Logical Operator13/1
  Logical Operator13/1 -> Switch2/2
  [PhaseMoveFalg0_L] -> Logical Operator12/1
  [PhaseMoveFalg1_S] -> Logical Operator8/2
  Logical Operator11/1 -> Logical Operator10/2
  [PhaseMoveFalg0_S] -> Logical Operator11/1
  Logical Operator8/1 -> Logical Operator10/1
  Logical Operator10/1 -> Switch1/2
  [PhaseMoveFalg1_L] -> Logical Operator9/2
  [PhaseMoveFalg2_L] -> Switch3/2, Logical Operator9/1
  Constant10/1 -> Add5/3
  Constant9/1 -> Add4/3
  Mux4/1 -> [SamplePoint]
  Add5/1 -> Mux4/2  "SamplePoint2"
  Add4/1 -> Mux4/1  "SamplePoint1"
  Constant8/1 -> Add5/2, Add4/2
  Mux3/1 -> [DutyMPM]  "DutyMPM"
  Mux2/1 -> [DutyLPM]  "DutyLPM"
  Mux1/1 -> [DutySPM]  "DutySPM"
  Signal Copy/1 -> Mux3/1  "DutyMU"
  Signal Copy1/1 -> Mux3/2  "DutyMD"
  [DutyM] -> Signal Copy/1, Signal Copy1/1
  [DutyL] -> Subtract7/1, Add3/1
  [PhaseMove_L] -> Add3/2, Subtract7/2
  Add3/1 -> Mux2/1  "DutyLU"
  Subtract7/1 -> Mux2/2, Add5/1  "DutyLD"
  Subtract5/1 -> Mux1/2  "DutySD"
  Add2/1 -> Add4/1, Mux1/1  "DutySU"
  [PhaseMove_S] -> Subtract5/2, Add2/2
  [DutyS] -> Add2/1, Subtract5/1
  Demux/3 -> [DutyS], Subtract/2
  Demux/2 -> Subtract/1, Subtract1/2, [DutyM]
  Demux/1 -> Subtract1/1, [DutyL]
  Subtract6/1 -> Switch3/1
  Constant7/1 -> Subtract6/1
  [DutyL] -> Subtract6/2
  Switch3/1 -> Switch2/1
  [T2divid2] -> Switch3/3
  Constant6/1 -> Switch2/3
  Switch2/1 -> [PhaseMove_L]  "PhaseMove_L"
  Subtract4/1 -> Switch/1
  [T1divid2] -> Switch/3
  Switch1/1 -> [PhaseMove_S]  "PhaseMove_S"
  Constant4/1 -> Switch1/3
  Switch/1 -> Switch1/1
  [PhaseMoveFalg2_S] -> Switch/2, Logical Operator8/1
  [DutyS] -> Subtract4/1
  Constant3/1 -> Subtract4/2
  Logical Operator3/1 -> [PhaseMoveFalg2_S], Logical Operator1/3  "PhaseMoveFalg2_S"
  Mux/1 -> [SampleValid]
  Constant2/1 -> Subtract3/2
  [T2divid2] -> Relational Operator1/1, Gain1/1, Compare To Constant3/1
  Gain1/1 -> Compare To Constant4/1
  [DutyL] -> Subtract2/2
  Constant1/1 -> Subtract2/1
  Subtract2/1 -> Add1/1, Relational Operator1/2
  Compare To Constant4/1 -> Logical Operator4/1
  Relational Operator1/1 -> Logical Operator6/1, Logical Operator4/2
  Logical Operator4/1 -> Logical Operator5/2, [PhaseMoveFalg1_L]  "PhaseMoveFalg1_L"
  [T2divid2] -> Add1/2
  Add1/1 -> Compare To Constant5/1
  Logical Operator7/1 -> Logical Operator5/3, [PhaseMoveFalg2_L]  "PhaseMoveFalg2_L"
  Logical Operator6/1 -> Logical Operator7/1
  Compare To Constant5/1 -> Logical Operator7/2
  Compare To Constant3/1 -> Logical Operator5/1, [PhaseMoveFalg0_L], Logical Operator15/1
  Logical Operator5/1 -> Mux/2  "SampleValid2"
  Logical Operator1/1 -> Mux/1  "SampleValid1"
  Compare To Constant/1 -> Logical Operator1/1, [PhaseMoveFalg0_S], Logical Operator14/1
  Add/1 -> Compare To Constant2/1  "T1/2+T0/4-DutyMin"
  [T1divid2] -> Add/2
  Logical Operator/1 -> [PhaseMoveFalg1_S], Logical Operator1/2  "PhaseMoveFalg1_S"
  Relational Operator/1 -> Logical Operator2/1, Logical Operator/3
  Subtract3/1 -> Relational Operator/2, Add/1  "T0/4-DutyMin"
  [DutyS] -> Subtract3/1
  Gain/1 -> Compare To Constant1/1
  [T1divid2] -> Compare To Constant/1, Gain/1, Relational Operator/1
  Saturation/1 -> DutySVPWM/1  "DutySVPWM[6]"
  Mux5/1 -> Saturation/1
  [SampleValid] -> SampleValid/1
  [SamplePoint] -> SamplePoint/1
  Multiport Switch/1 -> Mux5/1  "DutyAPM[2]"
  Multiport Switch2/1 -> Mux5/3  "DutyCPM[2]"
  Multiport Switch1/1 -> Mux5/2  "DutyBPM[2]"
  Constant5/1 -> Multiport Switch2/5, Multiport Switch/5, Multiport Switch1/5
  [DutySPM] -> Multiport Switch/4, Multiport Switch2/4, Multiport Switch1/4
  [DutyMPM] -> Multiport Switch/3, Multiport Switch1/3, Multiport Switch2/3
  [DutyLPM] -> Multiport Switch/2, Multiport Switch1/2, Multiport Switch2/2
  [SectorN] -> Multiport Switch/1, Multiport Switch1/1, Multiport Switch2/1
  SectorN/1 -> [SectorN]
  Subtract1/1 -> [T2divid2]  "T2/2"
  Subtract/1 -> [T1divid2]  "T1/2"
  DutyLMS/1 -> Demux/1

== system BLAC_MotorCtrl_Math/Hardware_Sim/CurrentSample_Sim/ADCSample_Sim ==
  Sample_In : Inport
  Add : Sum
  Add1 : Sum
  Band-Limited White Noise : simulink/Sources/Band-Limited White Noise  Cov=[0.1]  Ts=0.1  seed=[23341]
  Constant : Constant
  Data Type Conversion : DataTypeConversion  OutDataTypeStr=single  RndMeth=Simplest  SaturateOnIntegerOverflow=off
  Gain : Gain
  Sample_Out : Outport
  wires:
  Data Type Conversion/1 -> Sample_Out/1
  Add/1 -> Gain/1
  Constant/1 -> Add/2
  Gain/1 -> Data Type Conversion/1
  Add1/1 -> Add/1
  Sample_In/1 -> Add1/1
  Band-Limited White Noise/1 -> Add1/2

== system BLAC_MotorCtrl_Math/Hardware_Sim/CurrentSample_Sim/PhaseCurrentSmaple ==
  SampleTrigger : Inport
  SRV_C : Inport  Port=2
  SRV_B : Inport  Port=3
  SRV_A : Inport  Port=4
  ShuntV : Inport  Port=5
  CurrentSmaple_1RS : Subsystem  VariantControl=MC_Hardware_Sample_CurrentType == 1
  CurrentSmaple_2RS : Subsystem  VariantControl=MC_Hardware_Sample_CurrentType == 2
  CurrentSmaple_3RS : Subsystem  VariantControl=MC_Hardware_Sample_CurrentType == 3
  CurrentSampleResult : Outport

== system BLAC_MotorCtrl_Math/Hardware_Sim/Subsystem/PhaseM ==
  Current Sensor2 : fl_lib/Electrical/Electrical Sensors/Current Sensor
  PS-Simulink Converter : nesl_utility/PS-Simulink Converter  PhysicalDomain=network_engine_domain  SubClassName=ps_output  LeftPortType=input  RightPortType=output  PseudoPeriodic=off  Frequencies=[]  VectorFormat=inherit  Unit=inherit  AffineConversion=off
  PS-Simulink Converter1 : nesl_utility/PS-Simulink Converter  PhysicalDomain=network_engine_domain  SubClassName=ps_output  LeftPortType=input  RightPortType=output  PseudoPeriodic=off  Frequencies=[]  VectorFormat=inherit  Unit=inherit  AffineConversion=off
  Resistor1 : ee_lib/Passive/Resistor  R=1 Ohm  enable_R_tol=ee.enum.toleranceApplication.none  R_tol=5  tol_distribution=ee.enum.toleranceDistribution.uniform  nSigma=4  enable_operating_limits=ee.enum.enable.no  operating_limit_action=ee.enum.passive.reportOpLim.warn  power_rating=1 W  max_working_voltage=100 V  noise_mode=ee.enum.sources.noise.Disabled  Tdevice=25 degC  sample_time=1e-3 s  repeatability=ee.enum.ic.repeatability.notRepeatable  user_seed=0  auto_seed=545404223  power_derating_T1=70 degC  power_derating_T2=155 degC  operating_temperature_range_vec=[-50, 150] degC  alpha=3.93e-3 1/K  Tmeas=25 degC  thermal_mass=100 J/K  temperature_specify=off  temperature_priority=High  temperature=298.15 K  temperature_nominal_specify=off  temperature_nominal_value=1  temperature_nominal_unit=K
  Voltage Sensor : fl_lib/Electrical/Electrical Sensors/Voltage Sensor
  PhaseInput : PMIOPort  Side=Left
  PhaseOut : PMIOPort  Port=2  Side=Right
  N : PMIOPort  Port=3  Side=Right
  PhaseCurrent : Outport
  PhaseVoltage : Outport  Port=2
  wires:
  PS-Simulink Converter/1 -> PhaseCurrent/1
  PS-Simulink Converter1/1 -> PhaseVoltage/1
  connections:
  Resistor1/RConn1 -- Voltage Sensor/RConn2 -- N/RConn1
  Voltage Sensor/LConn1 -- PhaseOut/RConn1 -- Current Sensor2/RConn2 -- Resistor1/LConn1
  PS-Simulink Converter1/LConn1 -- Voltage Sensor/RConn1
  PS-Simulink Converter/LConn1 -- Current Sensor2/RConn1
  Current Sensor2/LConn1 -- PhaseInput/RConn1

== system BLAC_MotorCtrl_Math/Hardware_Sim/Subsystem/PhaseM1 ==
  Current Sensor2 : fl_lib/Electrical/Electrical Sensors/Current Sensor
  PS-Simulink Converter : nesl_utility/PS-Simulink Converter  PhysicalDomain=network_engine_domain  SubClassName=ps_output  LeftPortType=input  RightPortType=output  PseudoPeriodic=off  Frequencies=[]  VectorFormat=inherit  Unit=inherit  AffineConversion=off
  PS-Simulink Converter1 : nesl_utility/PS-Simulink Converter  PhysicalDomain=network_engine_domain  SubClassName=ps_output  LeftPortType=input  RightPortType=output  PseudoPeriodic=off  Frequencies=[]  VectorFormat=inherit  Unit=inherit  AffineConversion=off
  Resistor1 : ee_lib/Passive/Resistor  R=1 Ohm  enable_R_tol=ee.enum.toleranceApplication.none  R_tol=5  tol_distribution=ee.enum.toleranceDistribution.uniform  nSigma=4  enable_operating_limits=ee.enum.enable.no  operating_limit_action=ee.enum.passive.reportOpLim.warn  power_rating=1 W  max_working_voltage=100 V  noise_mode=ee.enum.sources.noise.Disabled  Tdevice=25 degC  sample_time=1e-3 s  repeatability=ee.enum.ic.repeatability.notRepeatable  user_seed=0  auto_seed=4112460543  power_derating_T1=70 degC  power_derating_T2=155 degC  operating_temperature_range_vec=[-50, 150] degC  alpha=3.93e-3 1/K  Tmeas=25 degC  thermal_mass=100 J/K  temperature_specify=off  temperature_priority=High  temperature=298.15 K  temperature_nominal_specify=off  temperature_nominal_value=1  temperature_nominal_unit=K
  Voltage Sensor : fl_lib/Electrical/Electrical Sensors/Voltage Sensor
  PhaseInput : PMIOPort  Side=Left
  PhaseOut : PMIOPort  Port=2  Side=Right
  N : PMIOPort  Port=3  Side=Right
  PhaseCurrent : Outport
  PhaseVoltage : Outport  Port=2
  wires:
  PS-Simulink Converter/1 -> PhaseCurrent/1
  PS-Simulink Converter1/1 -> PhaseVoltage/1
  connections:
  N/RConn1 -- Resistor1/RConn1 -- Voltage Sensor/RConn2
  Resistor1/LConn1 -- Voltage Sensor/LConn1 -- PhaseOut/RConn1 -- Current Sensor2/RConn2
  PS-Simulink Converter1/LConn1 -- Voltage Sensor/RConn1
  PS-Simulink Converter/LConn1 -- Current Sensor2/RConn1
  Current Sensor2/LConn1 -- PhaseInput/RConn1

== system BLAC_MotorCtrl_Math/Hardware_Sim/Subsystem/PhaseM2 ==
  Current Sensor2 : fl_lib/Electrical/Electrical Sensors/Current Sensor
  PS-Simulink Converter : nesl_utility/PS-Simulink Converter  PhysicalDomain=network_engine_domain  SubClassName=ps_output  LeftPortType=input  RightPortType=output  PseudoPeriodic=off  Frequencies=[]  VectorFormat=inherit  Unit=inherit  AffineConversion=off
  PS-Simulink Converter1 : nesl_utility/PS-Simulink Converter  PhysicalDomain=network_engine_domain  SubClassName=ps_output  LeftPortType=input  RightPortType=output  PseudoPeriodic=off  Frequencies=[]  VectorFormat=inherit  Unit=inherit  AffineConversion=off
  Resistor1 : ee_lib/Passive/Resistor  R=1 Ohm  enable_R_tol=ee.enum.toleranceApplication.none  R_tol=5  tol_distribution=ee.enum.toleranceDistribution.uniform  nSigma=4  enable_operating_limits=ee.enum.enable.no  operating_limit_action=ee.enum.passive.reportOpLim.warn  power_rating=1 W  max_working_voltage=100 V  noise_mode=ee.enum.sources.noise.Disabled  Tdevice=25 degC  sample_time=1e-3 s  repeatability=ee.enum.ic.repeatability.notRepeatable  user_seed=0  auto_seed=4144164703  power_derating_T1=70 degC  power_derating_T2=155 degC  operating_temperature_range_vec=[-50, 150] degC  alpha=3.93e-3 1/K  Tmeas=25 degC  thermal_mass=100 J/K  temperature_specify=off  temperature_priority=High  temperature=298.15 K  temperature_nominal_specify=off  temperature_nominal_value=1  temperature_nominal_unit=K
  Voltage Sensor : fl_lib/Electrical/Electrical Sensors/Voltage Sensor
  PhaseInput : PMIOPort  Side=Left
  PhaseOut : PMIOPort  Port=2  Side=Right
  N : PMIOPort  Port=3  Side=Right
  PhaseCurrent : Outport
  PhaseVoltage : Outport  Port=2
  wires:
  PS-Simulink Converter/1 -> PhaseCurrent/1
  PS-Simulink Converter1/1 -> PhaseVoltage/1
  connections:
  N/RConn1 -- Resistor1/RConn1 -- Voltage Sensor/RConn2
  Resistor1/LConn1 -- Voltage Sensor/LConn1 -- PhaseOut/RConn1 -- Current Sensor2/RConn2
  PS-Simulink Converter1/LConn1 -- Voltage Sensor/RConn1
  PS-Simulink Converter/LConn1 -- Current Sensor2/RConn1
  Current Sensor2/LConn1 -- PhaseInput/RConn1

== system BLAC_MotorCtrl_Math/Hardware_Sim/VbusSample_Sim/ADCSample_Sim ==
  Sample_In : Inport
  Trigger : TriggerPort  VariantControl=(inherit)  InitialTriggerSignalState=zero  PortDimensions=1
  Add : Sum
  Constant : Constant  Value=MC_Hardware_Chip_ADCVoltageRefence
  Data Type Conversion : DataTypeConversion  OutDataTypeStr=single  RndMeth=Simplest  SaturateOnIntegerOverflow=off
  Gain : Gain  Gain=2^(MC_Hardware_Chip_ADCResultBit)/MC_Hardware_Chip_ADCVoltageMax
  Sample_Out : Outport
  wires:
  Data Type Conversion/1 -> Sample_Out/1
  Constant/1 -> Add/2
  Sample_In/1 -> Add/1
  Add/1 -> Gain/1
  Gain/1 -> Data Type Conversion/1

== system BLAC_MotorCtrl_Math/Hardware_Sim/VbusSample_Sim/ADCSample_Sim1 ==
  Sample_In : Inport
  Trigger : TriggerPort  VariantControl=(inherit)  InitialTriggerSignalState=zero  PortDimensions=1
  Add : Sum
  Constant : Constant  Value=MC_Hardware_Chip_ADCVoltageRefence
  Data Type Conversion : DataTypeConversion  OutDataTypeStr=single  RndMeth=Simplest  SaturateOnIntegerOverflow=off
  Gain : Gain  Gain=2^(MC_Hardware_Chip_ADCResultBit)/MC_Hardware_Chip_ADCVoltageMax
  Sample_Out : Outport
  wires:
  Data Type Conversion/1 -> Sample_Out/1
  Constant/1 -> Add/2
  Sample_In/1 -> Add/1
  Add/1 -> Gain/1
  Gain/1 -> Data Type Conversion/1

== system BLAC_MotorCtrl_Math/HFTask/currentADRC/LESO/falFunc ==
  Err : Inport
  Alpha : Inport  Port=2
  Delta : Inport  Port=3
  Abs : Abs  SaturateOnIntegerOverflow=off
  Constant : Constant  OutDataTypeStr=single
  Divide : Product  Inputs=*/  OutDataTypeStr=single  RndMeth=Simplest
  Math Function : Math  Operator=pow  OutputSignalType=real
  Math Function1 : Math  Operator=pow  OutputSignalType=real
  Product : Product  OutDataTypeStr=single  RndMeth=Simplest
  Relational Operator : RelationalOperator  Operator=<=  OutDataTypeStr=boolean  RndMeth=Simplest  InputSameDT=off
  Sign : Signum
  Subtract : Sum  Inputs=+-
  Switch : Switch  Criteria=u2 > Threshold  SaturateOnIntegerOverflow=off  InputSameDT=off
  FalOutput : Outport
  wires:
  Switch/1 -> FalOutput/1
  Product/1 -> Switch/3
  Sign/1 -> Product/2
  Math Function1/1 -> Product/1
  Alpha/1 -> Subtract/2, Math Function1/2
  Divide/1 -> Switch/1
  Constant/1 -> Subtract/1
  Subtract/1 -> Math Function/2
  Math Function/1 -> Divide/2
  Relational Operator/1 -> Switch/2
  Delta/1 -> Relational Operator/2, Math Function/1
  Abs/1 -> Relational Operator/1, Math Function1/1
  Err/1 -> Abs/1, Sign/1, Divide/1

== system BLAC_MotorCtrl_Math/HFTask/svpwm/getVoltageExchange/getSectorN ==
  Valpha : Inport
  Vbeta : Inport  Port=2
  Add : Sum
  Add1 : Sum  Inputs=+++
  Constant : Constant
  Constant1 : Constant  Value=0
  Gain : Gain  Gain=sqrt(3)/2
  Gain1 : Gain  Gain=-1/2
  Gain2 : Gain
  Gain3 : Gain  Gain=2
  Gain4 : Gain  Gain=4
  Subtract : Sum  Inputs=-+
  Switch : Switch  Criteria=u2 > Threshold  SaturateOnIntegerOverflow=off  InputSameDT=off
  Switch1 : Switch  Criteria=u2 > Threshold  SaturateOnIntegerOverflow=off  InputSameDT=off
  Switch2 : Switch  Criteria=u2 > Threshold  SaturateOnIntegerOverflow=off  InputSameDT=off
  SectorN : Outport
  wires:
  Constant/1 -> Switch1/1, Switch/1, Switch2/1
  Gain3/1 -> Add1/2
  Gain1/1 -> Add/2, Subtract/2
  Switch/1 -> Gain2/1
  Gain/1 -> Add/1, Subtract/1
  Switch1/1 -> Gain3/1
  Vbeta/1 -> Switch/2, Gain1/1  "U1"
  Constant1/1 -> Switch2/3, Switch1/3, Switch/3
  Valpha/1 -> Gain/1
  Subtract/1 -> Switch2/2  "U3"
  Gain2/1 -> Add1/3
  Switch2/1 -> Gain4/1
  Add/1 -> Switch1/2  "U2"
  Gain4/1 -> Add1/1
  Add1/1 -> SectorN/1  "SectorN"

== system BLAC_MotorCtrl_Math/Hardware_Sim/CurrentSample_Sim/PhaseCurrentSmaple/CurrentSmaple_1RS ==
  SampleTrigger : Inport
  SRV_A : Inport  Port=2
  SRV_B : Inport  Port=3
  SRV_C : Inport  Port=4
  ShuntV : Inport  Port=5
  ADCSample_Sim : Subsystem
  ADCSample_Sim1 : Subsystem
  Add4 : Sum
  Band-Limited White Noise3 : simulink/Sources/Band-Limited White Noise  Cov=MC_Sim_NoisePower_PhaseCurrent  Ts=MC_Sim_BaseStep  seed=[23341]
  Demux : Demux  Outputs=3
  Mux : Mux  Inputs=2
  Terminator{1..4} (4 alike) : Terminator
  CurrentSampleResult : Outport
  wires:
  SRV_C/1 -> Terminator1/1
  SampleTrigger/1 -> Demux/1
  Demux/2 -> ADCSample_Sim1/Trigger
  Demux/1 -> ADCSample_Sim/Trigger
  ADCSample_Sim/1(Sample_Out) -> Mux/1
  ADCSample_Sim1/1(Sample_Out) -> Mux/2
  Mux/1 -> CurrentSampleResult/1
  Band-Limited White Noise3/1 -> Add4/2
  ShuntV/1 -> Add4/1
  Demux/3 -> Terminator2/1
  SRV_B/1 -> Terminator3/1
  SRV_A/1 -> Terminator4/1
  Add4/1 -> ADCSample_Sim1/1(Sample_In), ADCSample_Sim/1(Sample_In)

== system BLAC_MotorCtrl_Math/Hardware_Sim/CurrentSample_Sim/PhaseCurrentSmaple/CurrentSmaple_2RS ==
  SampleTrigger : Inport
  SRV_A : Inport  Port=2
  SRV_B : Inport  Port=3
  SRV_C : Inport  Port=4
  ShuntV : Inport  Port=5
  ADCSample_Sim : Subsystem
  ADCSample_Sim1 : Subsystem
  ADCSample_Sim3 : Subsystem
  Add1 : Sum
  Add2 : Sum
  Add4 : Sum
  Band-Limited White Noise : simulink/Sources/Band-Limited White Noise  Cov=MC_Sim_NoisePower_PhaseCurrent  Ts=MC_Sim_BaseStep  seed=[24541]
  Band-Limited White Noise1 : simulink/Sources/Band-Limited White Noise  Cov=MC_Sim_NoisePower_PhaseCurrent  Ts=MC_Sim_BaseStep  seed=[23657]
  Band-Limited White Noise3 : simulink/Sources/Band-Limited White Noise  Cov=MC_Sim_NoisePower_PhaseCurrent  Ts=MC_Sim_BaseStep  seed=[23561]
  Demux : Demux  Outputs=3
  Mux : Mux  Inputs=3
  Terminator : Terminator
  Terminator1 : Terminator
  CurrentSampleResult : Outport
  wires:
  Add2/1 -> ADCSample_Sim1/1(Sample_In)
  SRV_B/1 -> Add2/1
  ShuntV/1 -> Add4/1
  Add4/1 -> ADCSample_Sim3/1(Sample_In)
  Band-Limited White Noise3/1 -> Add4/2
  Band-Limited White Noise1/1 -> Add2/2
  Add1/1 -> ADCSample_Sim/1(Sample_In)
  SRV_A/1 -> Add1/1
  Band-Limited White Noise/1 -> Add1/2
  Mux/1 -> CurrentSampleResult/1
  ADCSample_Sim3/1(Sample_Out) -> Mux/3
  ADCSample_Sim1/1(Sample_Out) -> Mux/2
  ADCSample_Sim/1(Sample_Out) -> Mux/1
  Demux/3 -> ADCSample_Sim3/Trigger
  Demux/1 -> ADCSample_Sim1/Trigger, ADCSample_Sim/Trigger
  Demux/2 -> Terminator/1
  SampleTrigger/1 -> Demux/1
  SRV_C/1 -> Terminator1/1

== system BLAC_MotorCtrl_Math/Hardware_Sim/CurrentSample_Sim/PhaseCurrentSmaple/CurrentSmaple_3RS ==
  SampleTrigger : Inport
  SRV_A : Inport  Port=2
  SRV_B : Inport  Port=3
  SRV_C : Inport  Port=4
  ShuntV : Inport  Port=5
  ADCSample_Sim : Subsystem
  ADCSample_Sim1 : Subsystem
  ADCSample_Sim2 : Subsystem
  ADCSample_Sim3 : Subsystem
  Add{1..4} (4 alike) : Sum
  Band-Limited White Noise : simulink/Sources/Band-Limited White Noise  Cov=MC_Sim_NoisePower_PhaseCurrent  Ts=MC_Sim_BaseStep  seed=[2332]
  Band-Limited White Noise1 : simulink/Sources/Band-Limited White Noise  Cov=MC_Sim_NoisePower_PhaseCurrent  Ts=MC_Sim_BaseStep  seed=[23342]
  Band-Limited White Noise2 : simulink/Sources/Band-Limited White Noise  Cov=MC_Sim_NoisePower_PhaseCurrent  Ts=MC_Sim_BaseStep  seed=[22341]
  Band-Limited White Noise3 : simulink/Sources/Band-Limited White Noise  Cov=MC_Sim_NoisePower_PhaseCurrent  Ts=MC_Sim_BaseStep  seed=[24576]
  Demux : Demux  Outputs=3
  Mux : Mux
  Terminator : Terminator
  CurrentSampleResult : Outport
  wires:
  SampleTrigger/1 -> Demux/1
  Demux/2 -> Terminator/1
  Demux/1 -> ADCSample_Sim/Trigger, ADCSample_Sim2/Trigger, ADCSample_Sim1/Trigger
  Demux/3 -> ADCSample_Sim3/Trigger
  ADCSample_Sim/1(Sample_Out) -> Mux/1
  ADCSample_Sim1/1(Sample_Out) -> Mux/2
  ADCSample_Sim2/1(Sample_Out) -> Mux/3
  ADCSample_Sim3/1(Sample_Out) -> Mux/4
  Mux/1 -> CurrentSampleResult/1
  Band-Limited White Noise/1 -> Add1/2
  SRV_A/1 -> Add1/1
  Add1/1 -> ADCSample_Sim/1(Sample_In)
  Band-Limited White Noise1/1 -> Add2/2
  Band-Limited White Noise2/1 -> Add3/2
  Band-Limited White Noise3/1 -> Add4/2
  Add4/1 -> ADCSample_Sim3/1(Sample_In)
  ShuntV/1 -> Add4/1
  SRV_C/1 -> Add3/1
  SRV_B/1 -> Add2/1
  Add2/1 -> ADCSample_Sim1/1(Sample_In)
  Add3/1 -> ADCSample_Sim2/1(Sample_In)

== system BLAC_MotorCtrl_Math/Hardware_Sim/CurrentSample_Sim/PhaseCurrentSmaple/CurrentSmaple_1RS/ADCSample_Sim ==
  Sample_In : Inport
  Trigger : TriggerPort  VariantControl=(inherit)  PortDimensions=1
  Add : Sum
  Constant : Constant  Value=MC_Hardware_Chip_ADCVoltageRefence
  Data Type Conversion : DataTypeConversion  OutDataTypeStr=single  RndMeth=Simplest  SaturateOnIntegerOverflow=off
  Gain : Gain  Gain=2^(MC_Hardware_Chip_ADCResultBit)/MC_Hardware_Chip_ADCVoltageMax
  Gain1 : Gain  Gain=MC_Hardware_Chip_CSAGain
  Sample_Out : Outport
  wires:
  Data Type Conversion/1 -> Sample_Out/1
  Add/1 -> Gain/1
  Constant/1 -> Add/2
  Gain/1 -> Data Type Conversion/1
  Sample_In/1 -> Gain1/1
  Gain1/1 -> Add/1

== system BLAC_MotorCtrl_Math/Hardware_Sim/CurrentSample_Sim/PhaseCurrentSmaple/CurrentSmaple_1RS/ADCSample_Sim1 ==
  Sample_In : Inport
  Trigger : TriggerPort  TriggerType=falling  VariantControl=(inherit)  PortDimensions=1
  Add : Sum
  Constant : Constant  Value=MC_Hardware_Chip_ADCVoltageRefence
  Data Type Conversion : DataTypeConversion  OutDataTypeStr=single  RndMeth=Simplest  SaturateOnIntegerOverflow=off
  Gain : Gain  Gain=2^(MC_Hardware_Chip_ADCResultBit)/MC_Hardware_Chip_ADCVoltageMax
  Gain1 : Gain  Gain=MC_Hardware_Chip_CSAGain
  Sample_Out : Outport
  wires:
  Data Type Conversion/1 -> Sample_Out/1
  Constant/1 -> Add/2
  Add/1 -> Gain/1
  Gain/1 -> Data Type Conversion/1
  Sample_In/1 -> Gain1/1
  Gain1/1 -> Add/1

== system BLAC_MotorCtrl_Math/Hardware_Sim/CurrentSample_Sim/PhaseCurrentSmaple/CurrentSmaple_2RS/ADCSample_Sim ==
  Sample_In : Inport
  Trigger : TriggerPort  VariantControl=(inherit)  PortDimensions=1
  Add : Sum
  Constant : Constant  Value=MC_Hardware_Chip_ADCVoltageRefence
  Data Type Conversion : DataTypeConversion  OutDataTypeStr=single  RndMeth=Simplest  SaturateOnIntegerOverflow=off
  Gain : Gain  Gain=2^(MC_Hardware_Chip_ADCResultBit)/MC_Hardware_Chip_ADCVoltageMax
  Gain1 : Gain  Gain=MC_Hardware_Chip_CSAGain
  Sample_Out : Outport
  wires:
  Sample_In/1 -> Gain1/1
  Gain/1 -> Data Type Conversion/1
  Constant/1 -> Add/2
  Add/1 -> Gain/1
  Data Type Conversion/1 -> Sample_Out/1
  Gain1/1 -> Add/1

== system BLAC_MotorCtrl_Math/Hardware_Sim/CurrentSample_Sim/PhaseCurrentSmaple/CurrentSmaple_2RS/ADCSample_Sim1 ==
  Sample_In : Inport
  Trigger : TriggerPort  VariantControl=(inherit)  PortDimensions=1
  Add : Sum
  Constant : Constant  Value=MC_Hardware_Chip_ADCVoltageRefence
  Data Type Conversion : DataTypeConversion  OutDataTypeStr=single  RndMeth=Simplest  SaturateOnIntegerOverflow=off
  Gain : Gain  Gain=2^(MC_Hardware_Chip_ADCResultBit)/MC_Hardware_Chip_ADCVoltageMax
  Gain1 : Gain  Gain=MC_Hardware_Chip_CSAGain
  Sample_Out : Outport
  wires:
  Sample_In/1 -> Gain1/1
  Gain/1 -> Data Type Conversion/1
  Add/1 -> Gain/1
  Constant/1 -> Add/2
  Data Type Conversion/1 -> Sample_Out/1
  Gain1/1 -> Add/1

== system BLAC_MotorCtrl_Math/Hardware_Sim/CurrentSample_Sim/PhaseCurrentSmaple/CurrentSmaple_2RS/ADCSample_Sim3 ==
  Sample_In : Inport
  Trigger : TriggerPort  VariantControl=(inherit)  PortDimensions=1
  Add : Sum
  Constant : Constant  Value=MC_Hardware_Chip_ADCVoltageRefence
  Data Type Conversion : DataTypeConversion  OutDataTypeStr=single  RndMeth=Simplest  SaturateOnIntegerOverflow=off
  Gain : Gain  Gain=2^(MC_Hardware_Chip_ADCResultBit)/MC_Hardware_Chip_ADCVoltageMax
  Gain1 : Gain  Gain=MC_Hardware_Chip_CSAGain
  Sample_Out : Outport
  wires:
  Gain/1 -> Data Type Conversion/1
  Add/1 -> Gain/1
  Sample_In/1 -> Gain1/1
  Constant/1 -> Add/2
  Data Type Conversion/1 -> Sample_Out/1
  Gain1/1 -> Add/1

== system BLAC_MotorCtrl_Math/Hardware_Sim/CurrentSample_Sim/PhaseCurrentSmaple/CurrentSmaple_3RS/ADCSample_Sim ==
  Sample_In : Inport
  Trigger : TriggerPort  VariantControl=(inherit)  PortDimensions=1
  Add : Sum
  Constant : Constant  Value=MC_Hardware_Chip_ADCVoltageRefence
  Data Type Conversion : DataTypeConversion  OutDataTypeStr=single  RndMeth=Simplest  SaturateOnIntegerOverflow=off
  Gain : Gain  Gain=2^(MC_Hardware_Chip_ADCResultBit)/MC_Hardware_Chip_ADCVoltageMax
  Gain1 : Gain  Gain=MC_Hardware_Chip_CSAGain
  Sample_Out : Outport
  wires:
  Data Type Conversion/1 -> Sample_Out/1
  Add/1 -> Gain/1
  Constant/1 -> Add/2
  Gain/1 -> Data Type Conversion/1
  Sample_In/1 -> Gain1/1
  Gain1/1 -> Add/1

== system BLAC_MotorCtrl_Math/Hardware_Sim/CurrentSample_Sim/PhaseCurrentSmaple/CurrentSmaple_3RS/ADCSample_Sim1 ==
  Sample_In : Inport
  Trigger : TriggerPort  VariantControl=(inherit)  PortDimensions=1
  Add : Sum
  Constant : Constant  Value=MC_Hardware_Chip_ADCVoltageRefence
  Data Type Conversion : DataTypeConversion  OutDataTypeStr=single  RndMeth=Simplest  SaturateOnIntegerOverflow=off
  Gain : Gain  Gain=2^(MC_Hardware_Chip_ADCResultBit)/MC_Hardware_Chip_ADCVoltageMax
  Gain1 : Gain  Gain=MC_Hardware_Chip_CSAGain
  Sample_Out : Outport
  wires:
  Data Type Conversion/1 -> Sample_Out/1
  Constant/1 -> Add/2
  Add/1 -> Gain/1
  Gain/1 -> Data Type Conversion/1
  Sample_In/1 -> Gain1/1
  Gain1/1 -> Add/1

== system BLAC_MotorCtrl_Math/Hardware_Sim/CurrentSample_Sim/PhaseCurrentSmaple/CurrentSmaple_3RS/ADCSample_Sim2 ==
  Sample_In : Inport
  Trigger : TriggerPort  VariantControl=(inherit)  PortDimensions=1
  Add : Sum
  Constant : Constant  Value=MC_Hardware_Chip_ADCVoltageRefence
  Data Type Conversion : DataTypeConversion  OutDataTypeStr=single  RndMeth=Simplest  SaturateOnIntegerOverflow=off
  Gain : Gain  Gain=2^(MC_Hardware_Chip_ADCResultBit)/MC_Hardware_Chip_ADCVoltageMax
  Gain1 : Gain  Gain=MC_Hardware_Chip_CSAGain
  Sample_Out : Outport
  wires:
  Data Type Conversion/1 -> Sample_Out/1
  Constant/1 -> Add/2
  Sample_In/1 -> Gain1/1
  Add/1 -> Gain/1
  Gain/1 -> Data Type Conversion/1
  Gain1/1 -> Add/1
